simulink model "ARC_DTm"  (R2025b)
settings: Solver=FixedStepAuto  StartTime=0.0  StopTime=10080  FixedStep=1  RelTol=1e-3
PreLoadFcn:
  | %For Preload, set the working path
  | modelFolder = fileparts(which(bdroot));
  | addpath(genpath(modelFolder));
StartFcn:
  | tic
StopFcn:
  | fprintf("Sim Time: %.02f min", toc/60)
values from neighbouring files (symbols this model uses):
  batteryScenario = p.batteryScenario    [RUNSIM_ParameterSweep.m]    (also in _RUNSIM_ParameterSweep.m)
  Electricity_SalePriceModifier = 50/100    (= 0.5)    [RUNSIM_ParameterSweep.m]    (also in _RUNSIM_ParameterSweep.m)
  LUT = LUT_load.gamLUT    [RUNSIM_ParameterSweep.m]    (also in _RUNSIM_ParameterSweep.m)
  minimum_UF_system_flow = 5833    [RUNSIM_ParameterSweep.m]    (also in _RUNSIM_ParameterSweep.m)
  PROS1_recoveryrate = 61    [RUNSIM_ParameterSweep.m]    (also in _RUNSIM_ParameterSweep.m)
  PROS2_recoveryrate = 62    [RUNSIM_ParameterSweep.m]    (also in _RUNSIM_ParameterSweep.m)
  ROstabilization_time = p.ROstabilization_time    [RUNSIM_ParameterSweep.m]    (also in _RUNSIM_ParameterSweep.m)
  solarModifier = maximum_solar_generation / 300    [RUNSIM_ParameterSweep.m]    (also in _RUNSIM_ParameterSweep.m)
  TSRO_recoveryrate = 51    [RUNSIM_ParameterSweep.m]    (also in _RUNSIM_ParameterSweep.m)
  UF_RecoveryRate = 96    [RUNSIM_ParameterSweep.m]    (also in _RUNSIM_ParameterSweep.m)
undefined symbols (not defined in the file or in its folder): A_PROS1, A_PROS2, A_TSRO, B_PROS1, B_PROS2, B_TSRO, BW_Max_Time, BW_Max_Vol_gal, CEB_Max_Time, CEB_Max_Vol_gal, CIP_Max_Time, E, FF, h, L, w
libraries: simulink x40
(part 11 of 11)

== matlab function ARC_DTm/TSRO_Pump_2/MATLAB Function1 ==
  data: Q_des input; h_des input; power output
function power  = query_pump(Q_des, h_des)
% QUERY_PUMP Find pump speed, power, and efficiency given flow and head
%MUST UPDATE the pump_data call
%
% Inputs:
%   Q_des     - Desired flow rate (gpm)
%   h_des     - Desired added head (ft)
%   pump_data - Struct for a single pump (e.g. pump.pump_A)
%
% Outputs:
%   power      - Interpolated power
%   total_eff  - Interpolated total efficiency (%)
%   totalPower - Power demand accounting for efficiency (power / total_eff / 100)

persistent pump_data Q_min h_min P_min
if isempty(pump_data)
    loaded = coder.load('Pumps\LookupTables.mat');
    pump_data = loaded.pump.tsro;
    Q_min = min(pump_data.Q_grid(:));
    h_min = min(pump_data.H_grid(:));

    P_min = interp2(pump_data.Q_grid, pump_data.H_grid, pump_data.power_grid, h_min, Q_min, 'linear');

end

%zero flow conditions not present in the existing dataset.
if Q_des <= .1 * Q_min
    power = 0;
    return
end

% Normal lookup
power = interp2(pump_data.Q_grid, pump_data.H_grid, ...
    pump_data.power_grid, Q_des, h_des, 'linear');

if isnan(power)
    power = 0;
    return

end

== stateflow chart ARC_DTm/UF Maintenance Coordinator/arhive/UF_Operation State_10/UF10_Maintenance State ==
  settings: sampleTime=1  executeAtInitialization=1
  note: Unit State Machine — FIFO Maintenance Dispatch
      | This chart controls a single filtration unit through four operational states: Standby, Running, Await_Maintenance, BW_Maintenance, and CEB_Maintenance.
      | The unit begins in Standby, awaiting a startup command from the central dispatcher. Once commanded on, it enters Running, where it operates normally and tracks cumulative downtime. If a maintenance request is triggered, the unit transitions to Await_Maintenance, remaining online until the dispatcher confirms it can be released.
      | Two maintenance sequences are supported. A Backwash (BW) is a fixed-duration event (4 timesteps). A Chemically Enhanced Backwash (CEB) is a stochastic event lasting between 30 and 90 timesteps, sampled from a uniform distribution at entry. CEB is always followed by a BW cycle.
      | Upon completion of maintenance, the unit returns to Standby and re-enters the startup queue at the back, consistent with FIFO dispatching logic.
  note: Unit_cmd = 1 for running, 0 for off.
  state Standby
    during:
    %Unit is off, but awaiting startup.
    unit_in_startup_queue = 1;
    unit_in_operation = 0;
    %Ensure that the maintenance resets are occuring.
    maintenance_completion_indicator = 0;
  state Running
    entry:
    %Reset downtime timer
    cycle_downtime = 0;
    during:
    %Unit on, not in maint queue.
    unit_in_operation = 1;
    unit_in_maint_queue = 0;
  state Await_standby
    %Unit , Enter maint Queue
    during:
    unit_in_operation = 0;
    unit_in_maint_queue = 1;
  state Await_maintenance
    %Unit stays on, Enter maint Queue
    during:
    unit_in_operation = 1;
    unit_in_maint_queue = 1;
  state CEB_Maintenance
    %Unit is in chemically enhanced backwash. After CEB, do BW.
    %At start, determine a maintenance time within a uniform range of 30-60 min.
    entry:
    needed_maint_time = 30 + (60-30) * rand();
    %Exit state when time in maintenance is >= expected time.
    during:
    unit_in_operation = -1; %unit in maintenance
    %update maintenance time every step.
    cycle_downtime = cycle_downtime + 1;
  state BW_Maintenance
    entry:
    needed_maint_time = 1.5;
    %Exit state when time in maintenance is >= expected time.
    during:
    unit_in_operation = -1; %unit in maintenance
    %update maintenance time every step.
    cycle_downtime = cycle_downtime + 1;
    %ensure that the CEB is not continually reseting.
    maintenance_completion_indicator = 0;
  note: Maintenance Completion Indicator represents a signal to reset the counters at the UF unit tracking backwash cycles (signal = 2) and time in operations (signal = 1). These are pulse signals that reset integrators.
  (default) -> Running
  Standby -> Running : [startup_cmd == 1]{unit_in_startup_queue = 0;}
  Running -> (junction 44) [order 2] : [standby_cmd == 1]
  Running -> Await_maintenance [order 1] : [maint_req ~=0]
  (junction 22) -> Standby
  Await_standby -> (junction 47) : [standby_cmd == 1 && maint_cmd == 1]
  (junction 47) -> (junction 11)
  (junction 44) -> Await_standby
  Await_maintenance -> (junction 11) [order 2] : [maint_req == 1 && maint_cmd == 1] {unit_in_maint_queue = 0;}
  (junction 11) -> BW_Maintenance
  Await_maintenance -> CEB_Maintenance [order 1] : [maint_req == 2 && maint_cmd ==1]
  CEB_Maintenance -> BW_Maintenance : [after(needed_maint_time, tick)]{maintenance_completion_indicator = 2;}
  BW_Maintenance -> (junction 22) : [after(needed_maint_time, tick)]
      | {maintenance_completion_indicator = 1;}
  data: maint_cmd input; maint_req input; standby_cmd input; startup_cmd input; unit_in_maint_queue output; unit_in_startup_queue output; cycle_downtime local; needed_maint_time local; unit_in_operation output; maintenance_completion_indicator output

== stateflow chart ARC_DTm/UF Maintenance Coordinator/arhive/UF_Operation State_2/UF2_Maintenance State ==
  settings: sampleTime=1  executeAtInitialization=1
  note: Unit State Machine — FIFO Maintenance Dispatch
      | This chart controls a single filtration unit through four operational states: Standby, Running, Await_Maintenance, BW_Maintenance, and CEB_Maintenance.
      | The unit begins in Standby, awaiting a startup command from the central dispatcher. Once commanded on, it enters Running, where it operates normally and tracks cumulative downtime. If a maintenance request is triggered, the unit transitions to Await_Maintenance, remaining online until the dispatcher confirms it can be released.
      | Two maintenance sequences are supported. A Backwash (BW) is a fixed-duration event (4 timesteps). A Chemically Enhanced Backwash (CEB) is a stochastic event lasting between 30 and 90 timesteps, sampled from a uniform distribution at entry. CEB is always followed by a BW cycle.
      | Upon completion of maintenance, the unit returns to Standby and re-enters the startup queue at the back, consistent with FIFO dispatching logic.
  note: Unit_cmd = 1 for running, 0 for off.
  state Standby
    during:
    %Unit is off, but awaiting startup.
    unit_in_startup_queue = 1;
    unit_in_operation = 0;
    %Ensure that the maintenance resets are occuring.
    maintenance_completion_indicator = 0;
  state Running
    entry:
    %Reset downtime timer
    cycle_downtime = 0;
    during:
    %Unit on, not in maint queue.
    unit_in_operation = 1;
    unit_in_maint_queue = 0;
  state Await_standby
    %Unit , Enter maint Queue
    during:
    unit_in_operation = 0;
    unit_in_maint_queue = 1;
  state Await_maintenance
    %Unit stays on, Enter maint Queue
    during:
    unit_in_operation = 1;
    unit_in_maint_queue = 1;
  state CEB_Maintenance
    %Unit is in chemically enhanced backwash. After CEB, do BW.
    %At start, determine a maintenance time within a uniform range of 30-60 min.
    entry:
    needed_maint_time = 30 + (60-30) * rand();
    %Exit state when time in maintenance is >= expected time.
    during:
    unit_in_operation = -1; %unit in maintenance
    %update maintenance time every step.
    cycle_downtime = cycle_downtime + 1;
  state BW_Maintenance
    entry:
    needed_maint_time = 1.5;
    %Exit state when time in maintenance is >= expected time.
    during:
    unit_in_operation = -1; %unit in maintenance
    %update maintenance time every step.
    cycle_downtime = cycle_downtime + 1;
    %ensure that the CEB is not continually reseting.
    maintenance_completion_indicator = 0;
  note: Maintenance Completion Indicator represents a signal to reset the counters at the UF unit tracking backwash cycles (signal = 2) and time in operations (signal = 1). These are pulse signals that reset integrators.
  (default) -> Running
  Standby -> Running : [startup_cmd == 1]{unit_in_startup_queue = 0;}
  Running -> (junction 44) [order 2] : [standby_cmd == 1]
  Running -> Await_maintenance [order 1] : [maint_req ~=0]
  (junction 22) -> Standby
  Await_standby -> (junction 47) : [standby_cmd == 1 && maint_cmd == 1]
  (junction 47) -> (junction 11)
  (junction 44) -> Await_standby
  Await_maintenance -> (junction 11) [order 2] : [maint_req == 1 && maint_cmd == 1] {unit_in_maint_queue = 0;}
  (junction 11) -> BW_Maintenance
  Await_maintenance -> CEB_Maintenance [order 1] : [maint_req == 2 && maint_cmd ==1]
  CEB_Maintenance -> BW_Maintenance : [after(needed_maint_time, tick)]{maintenance_completion_indicator = 2;}
  BW_Maintenance -> (junction 22) : [after(needed_maint_time, tick)]
      | {maintenance_completion_indicator = 1;}
  data: maint_cmd input; maint_req input; standby_cmd input; startup_cmd input; unit_in_maint_queue output; unit_in_startup_queue output; cycle_downtime local; needed_maint_time local; unit_in_operation output; maintenance_completion_indicator output

== matlab function ARC_DTm/UVAOP 1/MATLAB Function ==
  data: feedFlow_gpm input; powerKW output
function powerKW = UVAOP_Train1Power(feedFlow_gpm)
% Inference-only prediction using pretrained model net_1flow
% Looks in base workspace first; falls back to net_1flow.mat

%#codegen
coder.extrinsic('evalin','load','predict','class');

persistent mdl
powerKW = 0.0;   % seed output type/size for Simulink

if isempty(mdl)
    mdl = evalin('base','net_1flow');
end

% Predict
powerKW = mdl(feedFlow_gpm);
end

== stateflow chart ARC_DTm/UF Maintenance Coordinator/arhive/UF_Operation State_3/UF3_Maintenance State ==
  settings: sampleTime=1  executeAtInitialization=1
  note: Unit State Machine — FIFO Maintenance Dispatch
      | This chart controls a single filtration unit through four operational states: Standby, Running, Await_Maintenance, BW_Maintenance, and CEB_Maintenance.
      | The unit begins in Standby, awaiting a startup command from the central dispatcher. Once commanded on, it enters Running, where it operates normally and tracks cumulative downtime. If a maintenance request is triggered, the unit transitions to Await_Maintenance, remaining online until the dispatcher confirms it can be released.
      | Two maintenance sequences are supported. A Backwash (BW) is a fixed-duration event (4 timesteps). A Chemically Enhanced Backwash (CEB) is a stochastic event lasting between 30 and 90 timesteps, sampled from a uniform distribution at entry. CEB is always followed by a BW cycle.
      | Upon completion of maintenance, the unit returns to Standby and re-enters the startup queue at the back, consistent with FIFO dispatching logic.
  note: Unit_cmd = 1 for running, 0 for off.
  state Standby
    during:
    %Unit is off, but awaiting startup.
    unit_in_startup_queue = 1;
    unit_in_operation = 0;
    %Ensure that the maintenance resets are occuring.
    maintenance_completion_indicator = 0;
  state Running
    entry:
    %Reset downtime timer
    cycle_downtime = 0;
    during:
    %Unit on, not in maint queue.
    unit_in_operation = 1;
    unit_in_maint_queue = 0;
  state Await_standby
    %Unit , Enter maint Queue
    during:
    unit_in_operation = 0;
    unit_in_maint_queue = 1;
  state Await_maintenance
    %Unit stays on, Enter maint Queue
    during:
    unit_in_operation = 1;
    unit_in_maint_queue = 1;
  state CEB_Maintenance
    %Unit is in chemically enhanced backwash. After CEB, do BW.
    %At start, determine a maintenance time within a uniform range of 30-60 min.
    entry:
    needed_maint_time = 30 + (60-30) * rand();
    %Exit state when time in maintenance is >= expected time.
    during:
    unit_in_operation = -1; %unit in maintenance
    %update maintenance time every step.
    cycle_downtime = cycle_downtime + 1;
  state BW_Maintenance
    entry:
    needed_maint_time = 1.5;
    %Exit state when time in maintenance is >= expected time.
    during:
    unit_in_operation = -1; %unit in maintenance
    %update maintenance time every step.
    cycle_downtime = cycle_downtime + 1;
    %ensure that the CEB is not continually reseting.
    maintenance_completion_indicator = 0;
  note: Maintenance Completion Indicator represents a signal to reset the counters at the UF unit tracking backwash cycles (signal = 2) and time in operations (signal = 1). These are pulse signals that reset integrators.
  (default) -> Running
  Standby -> Running : [startup_cmd == 1]{unit_in_startup_queue = 0;}
  Running -> (junction 44) [order 2] : [standby_cmd == 1]
  Running -> Await_maintenance [order 1] : [maint_req ~=0]
  (junction 22) -> Standby
  Await_standby -> (junction 47) : [standby_cmd == 1 && maint_cmd == 1]
  (junction 47) -> (junction 11)
  (junction 44) -> Await_standby
  Await_maintenance -> (junction 11) [order 2] : [maint_req == 1 && maint_cmd == 1] {unit_in_maint_queue = 0;}
  (junction 11) -> BW_Maintenance
  Await_maintenance -> CEB_Maintenance [order 1] : [maint_req == 2 && maint_cmd ==1]
  CEB_Maintenance -> BW_Maintenance : [after(needed_maint_time, tick)]{maintenance_completion_indicator = 2;}
  BW_Maintenance -> (junction 22) : [after(needed_maint_time, tick)]
      | {maintenance_completion_indicator = 1;}
  data: maint_cmd input; maint_req input; standby_cmd input; startup_cmd input; unit_in_maint_queue output; unit_in_startup_queue output; cycle_downtime local; needed_maint_time local; unit_in_operation output; maintenance_completion_indicator output

== stateflow chart ARC_DTm/UF Maintenance Coordinator/arhive/UF_Operation State_4/UF4_Maintenance State ==
  settings: sampleTime=1  executeAtInitialization=1
  note: Unit State Machine — FIFO Maintenance Dispatch
      | This chart controls a single filtration unit through four operational states: Standby, Running, Await_Maintenance, BW_Maintenance, and CEB_Maintenance.
      | The unit begins in Standby, awaiting a startup command from the central dispatcher. Once commanded on, it enters Running, where it operates normally and tracks cumulative downtime. If a maintenance request is triggered, the unit transitions to Await_Maintenance, remaining online until the dispatcher confirms it can be released.
      | Two maintenance sequences are supported. A Backwash (BW) is a fixed-duration event (4 timesteps). A Chemically Enhanced Backwash (CEB) is a stochastic event lasting between 30 and 90 timesteps, sampled from a uniform distribution at entry. CEB is always followed by a BW cycle.
      | Upon completion of maintenance, the unit returns to Standby and re-enters the startup queue at the back, consistent with FIFO dispatching logic.
  note: Unit_cmd = 1 for running, 0 for off.
  state Standby
    during:
    %Unit is off, but awaiting startup.
    unit_in_startup_queue = 1;
    unit_in_operation = 0;
    %Ensure that the maintenance resets are occuring.
    maintenance_completion_indicator = 0;
  state Running
    entry:
    %Reset downtime timer
    cycle_downtime = 0;
    during:
    %Unit on, not in maint queue.
    unit_in_operation = 1;
    unit_in_maint_queue = 0;
  state Await_standby
    %Unit , Enter maint Queue
    during:
    unit_in_operation = 0;
    unit_in_maint_queue = 1;
  state Await_maintenance
    %Unit stays on, Enter maint Queue
    during:
    unit_in_operation = 1;
    unit_in_maint_queue = 1;
  state CEB_Maintenance
    %Unit is in chemically enhanced backwash. After CEB, do BW.
    %At start, determine a maintenance time within a uniform range of 30-60 min.
    entry:
    needed_maint_time = 30 + (60-30) * rand();
    %Exit state when time in maintenance is >= expected time.
    during:
    unit_in_operation = -1; %unit in maintenance
    %update maintenance time every step.
    cycle_downtime = cycle_downtime + 1;
  state BW_Maintenance
    entry:
    needed_maint_time = 1.5;
    %Exit state when time in maintenance is >= expected time.
    during:
    unit_in_operation = -1; %unit in maintenance
    %update maintenance time every step.
    cycle_downtime = cycle_downtime + 1;
    %ensure that the CEB is not continually reseting.
    maintenance_completion_indicator = 0;
  note: Maintenance Completion Indicator represents a signal to reset the counters at the UF unit tracking backwash cycles (signal = 2) and time in operations (signal = 1). These are pulse signals that reset integrators.
  (default) -> Running
  Standby -> Running : [startup_cmd == 1]{unit_in_startup_queue = 0;}
  Running -> (junction 44) [order 2] : [standby_cmd == 1]
  Running -> Await_maintenance [order 1] : [maint_req ~=0]
  (junction 22) -> Standby
  Await_standby -> (junction 47) : [standby_cmd == 1 && maint_cmd == 1]
  (junction 47) -> (junction 11)
  (junction 44) -> Await_standby
  Await_maintenance -> (junction 11) [order 2] : [maint_req == 1 && maint_cmd == 1] {unit_in_maint_queue = 0;}
  (junction 11) -> BW_Maintenance
  Await_maintenance -> CEB_Maintenance [order 1] : [maint_req == 2 && maint_cmd ==1]
  CEB_Maintenance -> BW_Maintenance : [after(needed_maint_time, tick)]{maintenance_completion_indicator = 2;}
  BW_Maintenance -> (junction 22) : [after(needed_maint_time, tick)]
      | {maintenance_completion_indicator = 1;}
  data: maint_cmd input; maint_req input; standby_cmd input; startup_cmd input; unit_in_maint_queue output; unit_in_startup_queue output; cycle_downtime local; needed_maint_time local; unit_in_operation output; maintenance_completion_indicator output

== matlab function ARC_DTm/UVAOP 2/MATLAB Function ==
  data: feedFlow_gpm input; powerKW output
function powerKW = UVAOP_Train2Power(feedFlow_gpm)
% Inference-only prediction using pretrained model net_2flow
% Looks in base workspace first; falls back to net_2flow.mat

%#codegen
coder.extrinsic('evalin','load','predict','class');

persistent mdl
powerKW = 0.0;   % seed output type/size for Simulink

if isempty(mdl)
    mdl = evalin('base','net_2flow');
end

% Predict
powerKW = mdl(feedFlow_gpm);
end

== stateflow chart ARC_DTm/UF Maintenance Coordinator/arhive/UF_Operation State_5/UF5_Maintenance State ==
  settings: sampleTime=1  executeAtInitialization=1
  note: Unit State Machine — FIFO Maintenance Dispatch
      | This chart controls a single filtration unit through four operational states: Standby, Running, Await_Maintenance, BW_Maintenance, and CEB_Maintenance.
      | The unit begins in Standby, awaiting a startup command from the central dispatcher. Once commanded on, it enters Running, where it operates normally and tracks cumulative downtime. If a maintenance request is triggered, the unit transitions to Await_Maintenance, remaining online until the dispatcher confirms it can be released.
      | Two maintenance sequences are supported. A Backwash (BW) is a fixed-duration event (4 timesteps). A Chemically Enhanced Backwash (CEB) is a stochastic event lasting between 30 and 90 timesteps, sampled from a uniform distribution at entry. CEB is always followed by a BW cycle.
      | Upon completion of maintenance, the unit returns to Standby and re-enters the startup queue at the back, consistent with FIFO dispatching logic.
  note: Unit_cmd = 1 for running, 0 for off.
  state Standby
    during:
    %Unit is off, but awaiting startup.
    unit_in_startup_queue = 1;
    unit_in_operation = 0;
    %Ensure that the maintenance resets are occuring.
    maintenance_completion_indicator = 0;
  state Running
    entry:
    %Reset downtime timer
    cycle_downtime = 0;
    during:
    %Unit on, not in maint queue.
    unit_in_operation = 1;
    unit_in_maint_queue = 0;
  state Await_standby
    %Unit , Enter maint Queue
    during:
    unit_in_operation = 0;
    unit_in_maint_queue = 1;
  state Await_maintenance
    %Unit stays on, Enter maint Queue
    during:
    unit_in_operation = 1;
    unit_in_maint_queue = 1;
  state CEB_Maintenance
    %Unit is in chemically enhanced backwash. After CEB, do BW.
    %At start, determine a maintenance time within a uniform range of 30-60 min.
    entry:
    needed_maint_time = 30 + (60-30) * rand();
    %Exit state when time in maintenance is >= expected time.
    during:
    unit_in_operation = -1; %unit in maintenance
    %update maintenance time every step.
    cycle_downtime = cycle_downtime + 1;
  state BW_Maintenance
    entry:
    needed_maint_time = 1.5;
    %Exit state when time in maintenance is >= expected time.
    during:
    unit_in_operation = -1; %unit in maintenance
    %update maintenance time every step.
    cycle_downtime = cycle_downtime + 1;
    %ensure that the CEB is not continually reseting.
    maintenance_completion_indicator = 0;
  note: Maintenance Completion Indicator represents a signal to reset the counters at the UF unit tracking backwash cycles (signal = 2) and time in operations (signal = 1). These are pulse signals that reset integrators.
  (default) -> Running
  Standby -> Running : [startup_cmd == 1]{unit_in_startup_queue = 0;}
  Running -> (junction 44) [order 2] : [standby_cmd == 1]
  Running -> Await_maintenance [order 1] : [maint_req ~=0]
  (junction 22) -> Standby
  Await_standby -> (junction 47) : [standby_cmd == 1 && maint_cmd == 1]
  (junction 47) -> (junction 11)
  (junction 44) -> Await_standby
  Await_maintenance -> (junction 11) [order 2] : [maint_req == 1 && maint_cmd == 1] {unit_in_maint_queue = 0;}
  (junction 11) -> BW_Maintenance
  Await_maintenance -> CEB_Maintenance [order 1] : [maint_req == 2 && maint_cmd ==1]
  CEB_Maintenance -> BW_Maintenance : [after(needed_maint_time, tick)]{maintenance_completion_indicator = 2;}
  BW_Maintenance -> (junction 22) : [after(needed_maint_time, tick)]
      | {maintenance_completion_indicator = 1;}
  data: maint_cmd input; maint_req input; standby_cmd input; startup_cmd input; unit_in_maint_queue output; unit_in_startup_queue output; cycle_downtime local; needed_maint_time local; unit_in_operation output; maintenance_completion_indicator output
